simulink model "Vorlage_clamping_report"  (R2024a)
settings: Solver=ode45  StartTime=0.0  StopTime=1  FixedStep=1e-2  RelTol=1e-4  AbsTol=1e-4
values from neighbouring files (symbols this model uses):
  Kp = 9.8    [ITAE_Plots_PT2_limitations Rechenbeispiel.m]
  Td = 0.01    [ITAE_Plots_PT2_limitations Rechenbeispiel.m]
  Tf = 0.002    [ITAE_Plots_PT2_limitations Rechenbeispiel.m]
  Ti = 0.11    [ITAE_Plots_PT2_limitations Rechenbeispiel.m]
settings Model: Creator=bhir  LastModifiedBy=Flo
settings SolverCC: AlgebraicLoopSolver=TrustRegion
settings DataIOCC: ReturnWorkspaceOutputs=off
settings DebuggingCC: UnconnectedInputMsg=warning  UnconnectedOutputMsg=warning  UnconnectedLineMsg=warning  ArithmeticOperatorsInVariantConditions=warning
settings SFSimCC: SimUseLocalCustomCode=off  CustomCodeUndefinedFunction=UseInterfaceOnly
settings RTWCC: RTWUseLocalCustomCode=off  GPUComputeCapability=3.5  DLArmComputeVersion=19.05
settings CodeAppCC: StateflowObjectComments=on

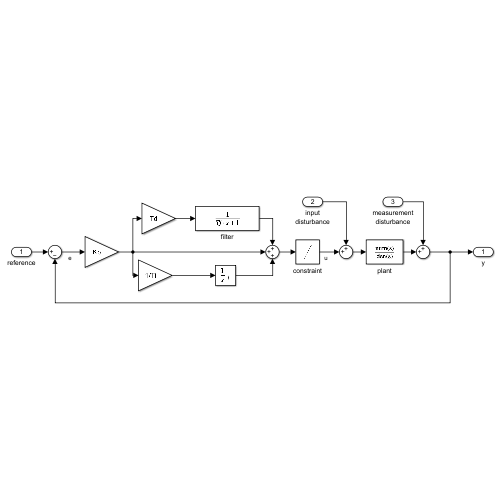
[thumbnail: Simulink's stored preview of the top-level diagram]
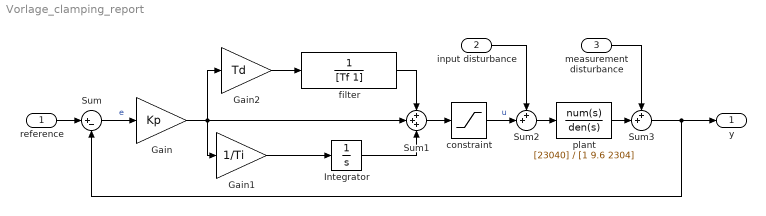
== system Vorlage_clamping_report ==
  reference : Inport
  input disturbance : Inport  Port=2
  measurement disturbance : Inport  Port=3
  Gain : Gain  Gain=Kp
  Gain1 : Gain  Gain=1/Ti
  Gain2 : Gain  Gain=Td
  Integrator : Integrator  LimitOutput=on
  Sum : Sum  Inputs=|+-
  Sum1 : Sum  Inputs=+++
  Sum2 : Sum  Inputs=++|
  Sum3 : Sum  Inputs=++|
  constraint : Saturate  UpperLimit=4  LowerLimit=-4
  filter : TransferFcn  Denominator=[Tf 1]
  plant : TransferFcn  Numerator=[23040]  Denominator=[1 9.6 2304]
  y : Outport
  wires:
  reference/1 -> Sum/1
  Sum/1 -> Gain/1  "e"
  Gain/1 -> Sum1/2, Gain2/1, Gain1/1
  filter/1 -> Sum1/1
  Gain2/1 -> filter/1
  Sum1/1 -> constraint/1
  Integrator/1 -> Sum1/3
  constraint/1 -> Sum2/2  "u"
  Sum2/1 -> plant/1
  plant/1 -> Sum3/2
  Sum3/1 -> y/1, Sum/2
  input disturbance/1 -> Sum2/1
  measurement disturbance/1 -> Sum3/1
  Gain1/1 -> Integrator/1
